simulink model "boost_converter"  (R2016a)
settings: Solver=FixedStepDiscrete  StartTime=0.0  StopTime=10  FixedStep=5e-6  RelTol=1e-3
libraries: powerlib x17, powerlib_meascontrol x1
settings Model: Creator=Dang Khoa  LastModifiedBy=Dang Khoa
settings GRTTargetCC: GeneratePreprocessorConditionals=Use local settings

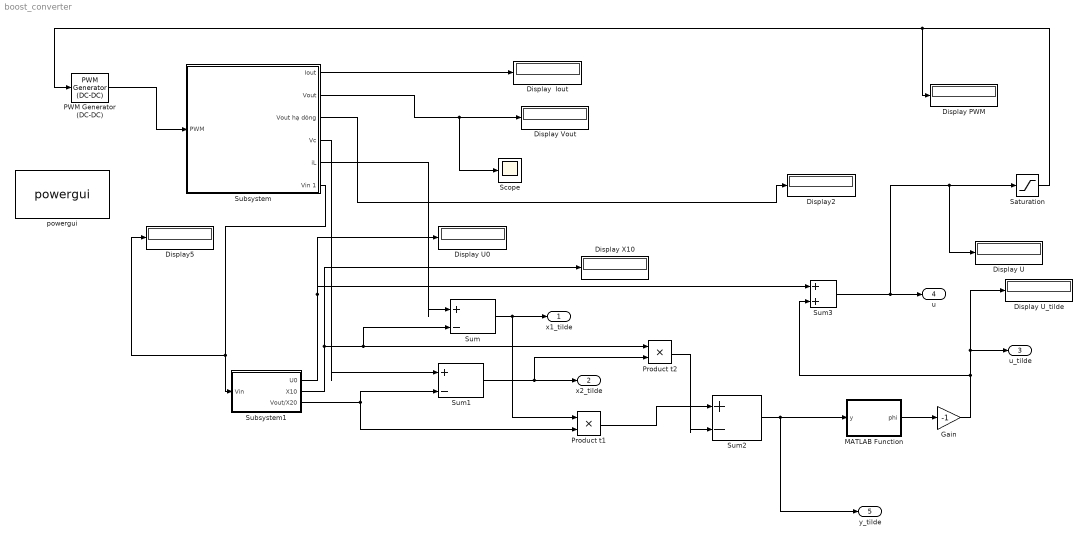
== system boost_converter ==
  Display  Iout : Display
  Display PWM : Display
  Display U : Display
  Display U0 : Display
  Display U_tilde : Display
  Display Vout : Display
  Display X10 : Display
  Display2 : Display
  Display5 : Display
  Gain : Gain  Gain=-1
  MATLAB Function : MATLAB Function  TreatAsAtomicUnit=on
  PWM Generator (DC-DC) : powerlib_meascontrol/Pulse & Signal Generators/PWM Generator (DC-DC)  Fsw=20000  Ts=5e-6
  Product t1 : Product
  Product t2 : Product
  Saturation : Saturate  UpperLimit=1  LowerLimit=0
  Scope : Scope
  Subsystem : Subsystem
  Subsystem1 : Subsystem
  Sum : Sum  Inputs=|+-
  Sum1 : Sum  Inputs=|+-
  Sum2 : Sum  Inputs=|+-
  Sum3 : Sum  Inputs=|++
  powergui : powerlib/powergui  Priority=1  SimulationMode=Discrete  SolverType=Tustin/Backward Euler (TBE)  SampleTime=5e-6  frequency=60  SPID=off  DisableSnubberDevices=off  DisableRonSwitches=off  DisableVfSwitches=off  SwTol=0  DisplayEquations=off  Interpol=off  ExternalGateDelay=off  methode=off  Ts=10  FunctionMessages=off  echomessages=off  HookPort=off  EnableUseOfTLC=off  x0status=blocks  frequencyindice=0  Pbase=100e6  ErrMax=1e-4  Iterations=50  UnitsV=kV  UnitsW=MW  buscounter=0  RestoreLinks=warning  ResistiveCurrentMeasurement=off  Frange=[0:2:500]  Ylog=off  Xlog=on  ShowGrid=off  save=off  variable=ZData  structure=0  ZoomFFT=off  StartTime=0.0  cycles=1  DisplayStyle=1  fundamental=60  FreqAxis=off  MaxFrequency=1000  frequencyindicesteady=1  RmsSteady=1  display=off
  x1_tilde : Outport
  x2_tilde : Outport  Port=2
  "u_tilde " : Outport  Port=3
  u : Outport  Port=4
  "y_tilde " : Outport  Port=5
  wires:
  Subsystem/1(Iout) -> Display  Iout/1
  Subsystem/2("Vout ") -> Scope/1, Display Vout/1
  Subsystem/3("Vout hạ dòng ") -> Display2/1
  PWM Generator (DC-DC)/1 -> Subsystem/1(PWM)
  Subsystem/5(iL) -> Sum/1
  Subsystem1/2("X10 ") -> Display X10/1, Product t2/1, Sum/2
  Sum/1 -> Product t1/1, x1_tilde/1
  Subsystem/4("Vc ") -> Sum1/1
  Subsystem1/3("Vout/X20 ") -> Product t1/2, Sum1/2
  Sum1/1 -> Product t2/2, x2_tilde/1
  Product t1/1 -> Sum2/1
  Product t2/1 -> Sum2/2
  MATLAB Function/1(phi) -> Gain/1
  Gain/1 -> Display U_tilde/1, "u_tilde "/1, Sum3/2
  Subsystem1/1(U0) -> Display U0/1, Sum3/1
  Subsystem/6(Vin 1) -> Display5/1, Subsystem1/1(Vin)
  Saturation/1 -> Display PWM/1, PWM Generator (DC-DC)/1
  Sum3/1 -> u/1, Display U/1, Saturation/1
  Sum2/1 -> MATLAB Function/1(y), "y_tilde "/1

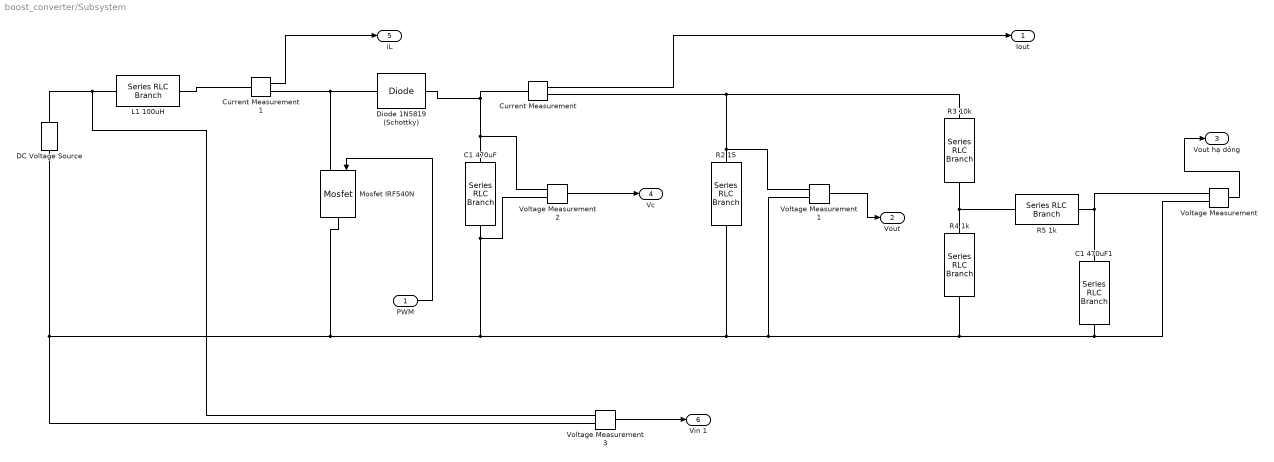
== system boost_converter/Subsystem ==
  PWM : Inport
  C1 470uF : powerlib/Elements/Series RLC Branch  LConnTagsString=__new0  RConnTagsString=__new0  BranchType=C  Resistance=1  Inductance=1e-3  SetiL0=off  InitialCurrent=0  Capacitance=470e-6  Setx0=off  InitialVoltage=0  Measurements=None
  C1 470uF1 : powerlib/Elements/Series RLC Branch  LConnTagsString=__new0  RConnTagsString=__new0  BranchType=C  Resistance=1  Inductance=1e-3  SetiL0=off  InitialCurrent=0  Capacitance=100e-9  Setx0=off  InitialVoltage=0  Measurements=None
  Current Measurement : powerlib/Measurements/Current Measurement  PhasorSimulation=off  OutputType=Complex  PSBequivalent=0
  Current Measurement1 : powerlib/Measurements/Current Measurement  PhasorSimulation=off  OutputType=Complex  PSBequivalent=0
  DC Voltage Source : powerlib/Electrical Sources/DC Voltage Source  Amplitude=15  Measurements=None
  Diode 1N5819 (Schottky) : powerlib/Power Electronics/Diode  Ron=0.05  Lon=0  Vf=0.45  IC=0  UseSnubber=off  Rs=500  Cs=250e-12  Measurements=off
  L1 100uH : powerlib/Elements/Series RLC Branch  LConnTagsString=__new0  RConnTagsString=__new0  BranchType=L  Resistance=1  Inductance=100e-6  SetiL0=off  InitialCurrent=0  Capacitance=1e-6  Setx0=off  InitialVoltage=0  Measurements=None
  Mosfet IRF540N : powerlib/Power Electronics/Mosfet  Ron=0.01  Lon=0  Rd=0.01  Vfd=0  IC=0  Rs=inf  Cs=inf  Measurements=off
  "R2 15 " : powerlib/Elements/Series RLC Branch  LConnTagsString=__new0  RConnTagsString=__new0  BranchType=R  Resistance=15  Inductance=1e-3  SetiL0=off  InitialCurrent=0  Capacitance=1e-6  Setx0=off  InitialVoltage=0  Measurements=None
  R3 10k : powerlib/Elements/Series RLC Branch  LConnTagsString=__new0  RConnTagsString=__new0  BranchType=R  Resistance=10000  Inductance=1e-3  SetiL0=off  InitialCurrent=0  Capacitance=1e-6  Setx0=off  InitialVoltage=0  Measurements=None
  R4 1k : powerlib/Elements/Series RLC Branch  LConnTagsString=__new0  RConnTagsString=__new0  BranchType=R  Resistance=1000  Inductance=1e-3  SetiL0=off  InitialCurrent=0  Capacitance=1e-6  Setx0=off  InitialVoltage=0  Measurements=None
  R5 1k : powerlib/Elements/Series RLC Branch  LConnTagsString=__new0  RConnTagsString=__new0  BranchType=R  Resistance=1000  Inductance=1e-3  SetiL0=off  InitialCurrent=0  Capacitance=1e-6  Setx0=off  InitialVoltage=0  Measurements=None
  Voltage Measurement{,1..3} (4 alike) : powerlib/Measurements/Voltage Measurement  PhasorSimulation=off  OutputType=Complex  PSBequivalent=0
  Iout : Outport
  "Vout " : Outport  Port=2
  "Vout hạ dòng " : Outport  Port=3
  "Vc " : Outport  Port=4
  iL : Outport  Port=5
  Vin 1 : Outport  Port=6
  wires:
  Current Measurement/1 -> Iout/1
  Voltage Measurement1/1 -> "Vout "/1
  Voltage Measurement/1 -> "Vout hạ dòng "/1
  PWM/1 -> Mosfet IRF540N/1
  Current Measurement1/1 -> iL/1
  Voltage Measurement2/1 -> "Vc "/1
  Voltage Measurement3/1 -> Vin 1/1
  connections:
  Mosfet IRF540N/LConn1 -- Current Measurement1/RConn1 -- Diode 1N5819 (Schottky)/LConn1
  DC Voltage Source/RConn1 -- Voltage Measurement3/LConn1 -- L1 100uH/LConn1
  Diode 1N5819 (Schottky)/RConn1 -- Voltage Measurement2/LConn1 -- C1 470uF/LConn1 -- Current Measurement/LConn1
  R4 1k/LConn1 -- R5 1k/LConn1 -- R3 10k/RConn1
  Voltage Measurement2/LConn2 -- C1 470uF/RConn1 -- Voltage Measurement1/LConn2 -- C1 470uF1/RConn1 -- Voltage Measurement/LConn2 -- R4 1k/RConn1 -- "R2 15 "/RConn1 -- Mosfet IRF540N/RConn1 -- Voltage Measurement3/LConn2 -- DC Voltage Source/LConn1
  "R2 15 "/LConn1 -- Current Measurement/RConn1 -- R3 10k/LConn1 -- Voltage Measurement1/LConn1
  R5 1k/RConn1 -- C1 470uF1/LConn1 -- Voltage Measurement/LConn1
  Current Measurement1/LConn1 -- L1 100uH/RConn1

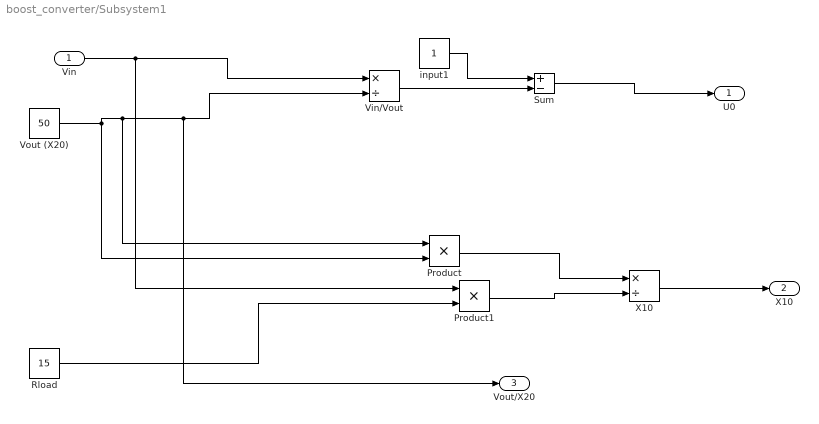
== system boost_converter/Subsystem1 ==
  Vin : Inport
  Product : Product
  Product1 : Product
  Rload : Constant  Value=15
  Sum : Sum  Inputs=+-
  "Vin/Vout " : Product  Inputs=*/
  "Vout (X20) " : Constant  Value=50
  X10 : Product  Inputs=*/
  input1 : Constant
  U0 : Outport
  "X10 " : Outport  Port=2
  "Vout/X20 " : Outport  Port=3
  wires:
  Sum/1 -> U0/1
  Rload/1 -> Product1/2
  Vin/1 -> "Vin/Vout "/1, Product1/1
  input1/1 -> Sum/1
  "Vin/Vout "/1 -> Sum/2
  "Vout (X20) "/1 -> Product/1, "Vout/X20 "/1, "Vin/Vout "/2, Product/2
  Product/1 -> X10/1
  Product1/1 -> X10/2
  X10/1 -> "X10 "/1

== matlab function boost_converter/MATLAB Function ==
  data: y input; phi output
function phi = PBCphi(y)
a1 = 1.0;   % đáp ứng chính
a2 = 0.10;  % chống lệch lớn
a3 = 0.015; % giảm rung quanh điểm đặt
phi = a1*y + a2*y^3 + a3*y^5;
